simulink model "MPCtest"  (Simulink 9.2)
settings: Solver=ode45  StartTime=0  StopTime=8  FixedStep=0.002  RelTol=1e-3  AbsTol=1e-6
InitFcn:
  | R2D = 180/pi;
libraries: Solver_SF x1, simulink x1
settings Model: Creator=jason  LastModifiedBy=jason  ExtModeTrigMode=oneshot  ExtModeArmWhenConnect=off
settings SolverCC: AutoScaleAbsTol=off
settings DataIOCC: LimitDataPoints=off  SignalLoggingName=sigsOut
settings OptimizationCC: BlockReduction=off  BooleanDataType=off  InitFltsAndDblsToZero=on
settings DebuggingCC: SaveWithParameterizedLinksMsg=none  SignalResolutionControl=TryResolveAllWithWarning  MultiTaskDSMMsg=warning  MultiTaskCondExecSysMsg=none  StateNameClashWarn=none
settings HardwareCC: TargetUnknown=on
settings SFSimCC: SimUseLocalCustomCode=on
settings RTWCC: TemplateMakefile=grt_vc.tmf  RTWUseLocalCustomCode=on
settings GRTTargetCC: TargetFcnLib=ansi_tfl_tmw.mat  GeneratePreprocessorConditionals=Use local settings
settings ConfigComp: CovExternalEMLEnable=on

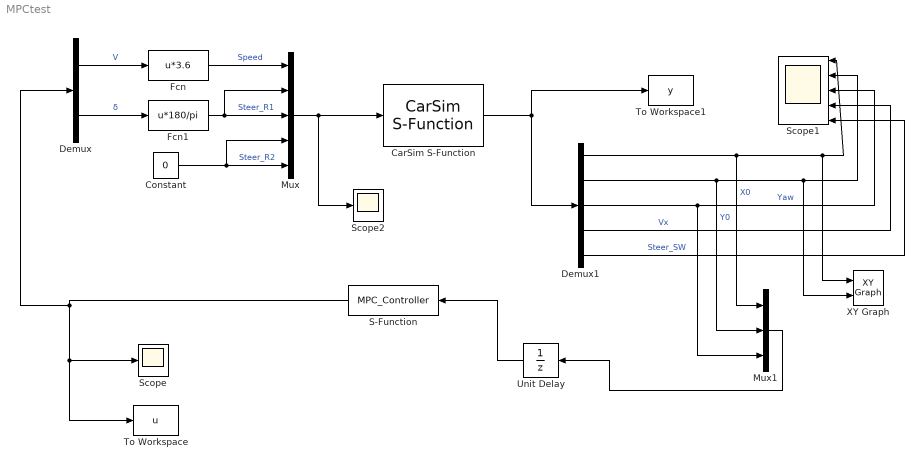
== system MPCtest ==
  CarSim S-Function : Solver_SF/CarSim S-Function  Priority=1  VehicleCode=i_i  SIMFILE=simfile
  Constant : Constant  Value=0
  Demux : Demux  Outputs=2
  Demux1 : Demux  Outputs=5
  Fcn : Fcn  Expr=u*3.6
  Fcn1 : Fcn  Expr=u*180/pi
  Mux : Mux  Inputs=5
  Mux1 : Mux  Inputs=3
  S-Function : S-Function  FunctionName=MPC_Controller  SFunctionDeploymentMode=off  EnableBusSupport=off
  Scope : Scope
  Scope1 : Scope  NumInputPorts=5
  Scope2 : Scope
  To Workspace : ToWorkspace  VariableName=u  SaveFormat=Timeseries  SampleTime=-1
  To Workspace1 : ToWorkspace  VariableName=y  SaveFormat=Timeseries  SampleTime=-1
  Unit Delay : UnitDelay  SampleTime=-1
  XY Graph : simulink/Sinks/XY Graph  xmin=-1  xmax=1  ymin=-1  ymax=1  st=-1
  wires:
  Mux/1 -> Scope2/1, CarSim S-Function/1
  Fcn/1 -> Mux/1  "Speed"
  Fcn1/1 -> Mux/3, Mux/2  "Steer_R1"
  Constant/1 -> Mux/5, Mux/4  "Steer_R2"
  Demux/1 -> Fcn/1  "V"
  Demux/2 -> Fcn1/1  "δ"
  S-Function/1 -> Scope/1, To Workspace/1, Demux/1
  Unit Delay/1 -> S-Function/1
  CarSim S-Function/1 -> Demux1/1, To Workspace1/1
  Demux1/1 -> Mux1/1, XY Graph/1, Scope1/1  "X0"
  Demux1/2 -> Mux1/2, XY Graph/2, Scope1/2  "Y0"
  Demux1/3 -> Mux1/3, Scope1/3  "Yaw"
  Demux1/4 -> Scope1/4  "Vx"
  Demux1/5 -> Scope1/5  "Steer_SW"
  Mux1/1 -> Unit Delay/1
